simulink model "linear_and_quad_sim"  (R2020a)
settings: Solver=FixedStepAuto  StartTime=0.0  StopTime=1.5  FixedStep=0.0001  RelTol=1e-3
undefined symbols (not defined in the file or in its folder): c, k, m, q
settings Model: Creator=User  LastModifiedBy=User

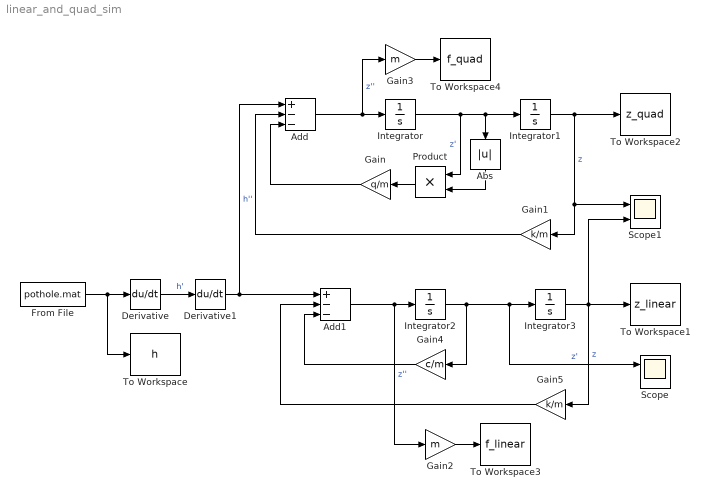
== system linear_and_quad_sim ==
  Abs : Abs
  Add : Sum  Inputs=+--
  Add1 : Sum  Inputs=+--
  Derivative : Derivative
  Derivative1 : Derivative
  From File : FromFile  FileName=pothole.mat
  Gain : Gain  Gain=q/m
  Gain1 : Gain  Gain=k/m
  Gain2 : Gain  Gain=m
  Gain3 : Gain  Gain=m
  Gain4 : Gain  Gain=c/m
  Gain5 : Gain  Gain=k/m
  Integrator{,1..3} (4 alike) : Integrator
  Product : Product
  Scope : Scope  NumInputPorts=2
  Scope1 : Scope  NumInputPorts=2
  To Workspace : ToWorkspace  VariableName=h  SampleTime=-1
      settings: Save2DSignal=2-D array (concatenate along first dimension)
  To Workspace1 : ToWorkspace  VariableName=z_linear  SampleTime=-1
      settings: Save2DSignal=2-D array (concatenate along first dimension)
  To Workspace2 : ToWorkspace  VariableName=z_quad  SampleTime=-1
      settings: Save2DSignal=2-D array (concatenate along first dimension)
  To Workspace3 : ToWorkspace  VariableName=f_linear  SampleTime=-1
      settings: Save2DSignal=2-D array (concatenate along first dimension)
  To Workspace4 : ToWorkspace  VariableName=f_quad  SampleTime=-1
      settings: Save2DSignal=2-D array (concatenate along first dimension)
  wires:
  Gain/1 -> Add/3
  Integrator/1 -> Abs/1, Integrator1/1, Product/1  "z'"
  Add/1 -> Gain3/1, Integrator/1  "z''"
  Product/1 -> Gain/1
  Integrator1/1 -> Gain1/1, Scope1/1, To Workspace2/1  "z"
  Gain1/1 -> Add/2
  Abs/1 -> Product/2
  Integrator3/1 -> Scope1/2, To Workspace1/1, Gain5/1  "z"
  Gain4/1 -> Add1/3
  Add1/1 -> Gain2/1, Integrator2/1  "z''"
  Integrator2/1 -> Gain4/1, Scope/1, Integrator3/1  "z'"
  Gain5/1 -> Add1/2
  Derivative/1 -> Derivative1/1  "h'"
  Derivative1/1 -> Add/1, Add1/1  "h''"
  From File/1 -> To Workspace/1, Derivative/1
  Gain2/1 -> To Workspace3/1
  Gain3/1 -> To Workspace4/1
